simulink model "BLDCmotorControl_FOC_R2017b_fixdt_Ffwd"  (R2017b)
settings: Solver=FixedStepDiscrete  StartTime=0  StopTime=0.5  FixedStep=Ts  MaxStep=1e-6  RelTol=1e-6  AbsTol=1e-6  EnableMultiTasking=on
PreLoadFcn:
  | addpath(genpath('01_Libraries'));
  | addpath(genpath('02_Figures'));
InitFcn:
  | init_model;
values from neighbouring files (symbols this model uses):
  a_elecAngle = 60    [init_model_Ffwd.m]
  b_DCLinkCurrAvail = 0    [init_model_Ffwd.m]
  b_diagEna = 1    [init_model_Ffwd.m]
  b_FfwdEna = 1    [init_model_Ffwd.m]
  b_fieldWeakEna = 0    [init_model_Ffwd.m]
  b_selPhaABCurrMeas = 1    [init_model_Ffwd.m]
  cf_currFilt = 0.02    [init_model_Ffwd.m]
  cf_speedCoef = round(f_ctrl * a_mechAngle * (pi/180) * (30/pi))    [init_model_Ffwd.m]
  cf_speedFilt = 0.20    (= 0.2)    [init_model_Ffwd.m]
  CTRL_COM = 0    [init_model_Ffwd.m]
  dV_openRate = 1000 * Ts_ctrl    (= 0.06)    [init_model_Ffwd.m]
  dz_cntTrnsDetHi = 40    [init_model_Ffwd.m]
  dz_cntTrnsDetLo = 20    [init_model_Ffwd.m]
  i_errThres = 40 * i_sca    (= 2000)    [init_model_Ffwd.m]
  i_max = i_max * i_sca    (= 750)    [init_model_Ffwd.m]
  i_thresOutlier = 200    [init_model_Ffwd.m]
  id_fieldWeak_M1 = [  0   0  0.05  0.25    1    2    3    4  4.5  4.8   5   5] * i_sca    [init_model_Ffwd.m]
  id_Kb = 1000 * Ts_ctrl    (= 0.06)    [init_model_Ffwd.m]
  id_Ki = 80 * Ts_ctrl    (= 0.0048)    [init_model_Ffwd.m]
  id_Kp = 0.5    [init_model_Ffwd.m]
  iq_Kb = 1000 * Ts_ctrl    (= 0.06)    [init_model_Ffwd.m]
  iq_Ki = 100 * Ts_ctrl    (= 0.006)    [init_model_Ffwd.m]
  iq_KiLimProt = 3 * Ts_ctrl    (= 0.00018)    [init_model_Ffwd.m]
  iq_Kp = 0.5    [init_model_Ffwd.m]
  iq_KpLimProt = 4    [init_model_Ffwd.m]
  iq_max_M1 = sqrt(i_max^2 - iq_max_XA.^2)    [init_model_Ffwd.m]
  Ld = 0.00024368    [pe_electric_engine_dyno_data.m]
  Lq = 0.00029758    [pe_electric_engine_dyno_data.m]
  mot_lambda = 0    [init_model_Ffwd.m]
  mot_Ld = 0    [init_model_Ffwd.m]
  mot_Lq = 0    [init_model_Ffwd.m]
  n_commAcvLo = 15    [init_model_Ffwd.m]
  n_commDeacvHi = 30    [init_model_Ffwd.m]
  n_Kb = 1000 * Ts_ctrl    (= 0.06)    [init_model_Ffwd.m]
  n_Ki = 10 * Ts_ctrl    (= 0.0006)    [init_model_Ffwd.m]
  n_Kp = 1    [init_model_Ffwd.m]
  n_KpLimProt = 5    [init_model_Ffwd.m]
  n_max = 800    [init_model_Ffwd.m]
  n_stdStillDet = 3    [init_model_Ffwd.m]
  OPEN_MODE = 0    [init_model_Ffwd.m]
  r_cos_M1 = cos((a_elecAngle_XA + 30)*(pi/180))    [init_model_Ffwd.m]
  r_sin_M1 = sin((a_elecAngle_XA + 30)*(pi/180))    [init_model_Ffwd.m]
  r_whl = 6.5 * 2.54 * 1e-2 / 2    (= 0.08255)    [init_model_Ffwd.m]
  Rs = 0.010087    [pe_electric_engine_dyno_data.m]
  SPD_MODE = 2    [init_model_Ffwd.m]
  t_errDequal = 2 * f_ctrl    (= 32000)    [init_model_Ffwd.m]
  t_errQual = 0.8 * f_ctrl    (= 12800)    [init_model_Ffwd.m]
  TRQ_MODE = 3    [init_model_Ffwd.m]
  Ts = 5e-6    (= 5e-06)    [init_model_Ffwd.m]    (also in pe_electric_engine_dyno_data.m = 1e-05)
  Ts_ctrl = 6e-5    (= 6e-05)    [init_model_Ffwd.m]
  Vd_max = 1000 - V_margin    (= 900)    [init_model_Ffwd.m]
  vec_hallToPos = [0 2 0 1 4 3 5 0]    [init_model_Ffwd.m]
  VLT_MODE = 1    [init_model_Ffwd.m]
  Vq_max_M1 = sqrt(Vd_max^2 - Vq_max_XA.^2)    [init_model_Ffwd.m]
  z_commutMap_M1 = [-1 -1  0  1  1  0 ... (first row only)    [init_model_Ffwd.m]
  z_ctrlModReq = 1    [init_model_Ffwd.m]
  z_ctrlTypSel = 1    [init_model_Ffwd.m]
  z_maxCntRst = 2000    [init_model_Ffwd.m]
undefined symbols (not defined in the file or in its folder): DiscIntNeverNeededParam, sigbuilder_block, V_max, V_min
libraries: powerlib x14, BLDC_controller_Lib x12, simulink x11, pePwmGenerator x1
(part 1 of 3)
Description:
  | This model implements FOC controller for a BLDC motor.
  | The controller is capable for embedded code generation.
  | 
  | Copyright © 2019 Emanuel FERU
settings Model: ExtModeAutoUpdateStatusClock=off  TunableVars=Vd_max,Vq_max_M1,Vq_max_XA,b_DCLinkCurrAvail,b_diagEna,b_fieldWeakEna,b_selPhaABCurrMeas,cf_currFilt,cf_speedCoef,cf_speedFilt,dV_openRate,dz_cntTrnsDetHi,dz_cntTrnsDetLo,i_errThres,i_max,i_thresOutlier,id_Kb,id_Ki,id_Kp,id_fieldWeak_M1,iq_Kb,iq_Ki,iq_KiLimProt,iq_Kp,iq_KpLimProt,iq_max_M1,iq_max_XA,mot_Ld,mot_Lq,mot_lambda,n_Kb,n_Ki,n_Kp,n_KpLimProt,n_commAcvLo,n_commDeacvHi,n_fieldWeak_XA,n_max,n_stdStillDet,t_errDequal,t_errQual,z_ctrlModReq,z_ctrlTypSel,z_maxCntRst  TunableVarsStorageClass=Auto,Auto,Auto,Auto,Auto,Auto,Auto,Auto,Auto,Auto,Auto,Auto,Auto,Auto,Auto,Auto,Auto,Auto,Auto,Auto,Auto,Auto,Auto,Auto,Auto,Auto,Auto,Auto,Auto,Auto,Auto,Auto,Auto,Auto,Auto,Auto,Auto,Auto,Auto,Auto,Auto,Auto,Auto,Auto  TunableVarsTypeQualifier=,,,,,,,,,,,,,,,,,,,,,,,,,,,,,,,,,,,,,,,,,,,  Creator=MathWorks  LastModifiedBy=eferu
settings SolverCC: AutoInsertRateTranBlk=on
settings DataIOCC: LimitDataPoints=on  SaveFormat=Array  ReturnWorkspaceOutputs=on  SignalLoggingName=sigsOut
settings OptimizationCC: DefaultParameterBehavior=Inlined  UseDivisionForNetSlopeComputation=on  UseFloatMulNetSlope=on  UseSpecifiedMinMax=on  InlineInvariantSignals=on  PassReuseOutputArgsAs=Individual arguments  ExpressionDepthLimit=2147483647  ZeroExternalMemoryAtStartup=off  ZeroInternalMemoryAtStartup=off  NoFixptDivByZeroProtection=on  EfficientFloat2IntCast=on  LifeSpan=1  OptimizeBlockOrder=speed  DifferentSizesBufferReuse=on
settings DebuggingCC: ReadBeforeWriteMsg=DisableAll  WriteAfterWriteMsg=DisableAll  WriteAfterReadMsg=DisableAll  UnderspecifiedInitializationDetection=Classic  InheritedTsInSrcMsg=none  MultiTaskDSMMsg=none  MultiTaskCondExecSysMsg=none  ParameterTunabilityLossMsg=error  FcnCallInpInsideContextMsg=warning  StateNameClashWarn=warning  SFUnexpectedBacktrackingDiag=warning  SFNoUnconditionalDefaultTransitionDiag=warning  SFExecutionAtInitializationDiag=none
settings HardwareCC: ProdBitPerPointer=32  ProdBitPerSizeT=32  ProdBitPerPtrDiffT=32  ProdLargestAtomicInteger=Long  ProdLargestAtomicFloat=Double  ProdWordSize=32  ProdHWDeviceType=ARM Compatible->ARM Cortex  TargetUnknown=on
settings ModelReferenceCC: UpdateModelReferenceTargets=IfOutOfDate  PropagateSignalLabelsOutOfModel=off
settings SFSimCC: SFSimEcho=off  MATLABDynamicMemAlloc=off
settings RTWCC: SystemTargetFile=ert.tlc  GenCodeOnly=on  TemplateMakefile=ert_default_tmf  GenerateReport=on  BuildConfiguration=Faster Runs  IncludeHyperlinkInReport=on  LaunchReport=on  GenerateTraceInfo=on  GenerateTraceReport=on  GenerateTraceReportSl=on  GenerateTraceReportSf=on  GenerateTraceReportEml=on  GenerateCodeMetricsReport=on  GenerateCodeReplacementReport=on
settings CodeAppCC: ForceParamTrailComments=on  IgnoreCustomStorageClasses=off  OperatorAnnotations=on  SimulinkDataObjDesc=on  SFDataObjDesc=on  CustomSymbolStrGlobalVar=rt$N$M  CustomSymbolStrType=$N$M  CustomSymbolStrFcn=$N$M$F  CustomSymbolStrMacro=$N$M  InsertBlockDesc=on
settings ERTTargetCC: GenerateSampleERTMain=on  IncludeMdlTerminateFcn=off  CombineSignalStateStructs=on  SuppressErrorStatus=on  MultiInstanceERTCode=on  CodeInterfacePackaging=Reusable function  SupportNonFinite=off  SupportComplex=off  InlinedParameterPlacement=NonHierarchical  RootIOFormat=Part of model data structure  ERTCustomFileTemplate=example_file_process.tlc  ERTFilePackagingFormat=CompactWithDataFile  PreserveStaticInFcnDecls=off
settings ConfigComp: CovMetricSettings=dw  CovHtmlReporting=on  CovSaveCumulativeToWorkspaceVar=on  CovSaveSingleToWorkspaceVar=on  CovExternalEMLEnable=off  CovSFcnEnable=off
settings SimscapeCC: SimscapeNormalizeSystem=off

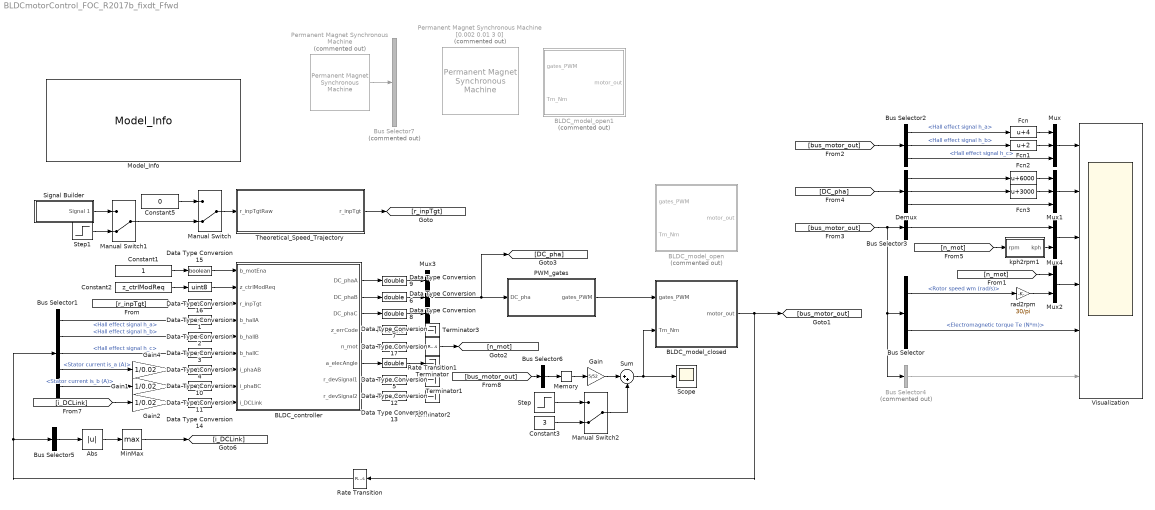
== system BLDCmotorControl_FOC_R2017b_fixdt_Ffwd ==
  Abs : Abs
  BLDC_controller : Subsystem  TreatAsAtomicUnit=on  SystemSampleTime=Ts_ctrl
  BLDC_model_closed : Subsystem
      mask help: Simulink:masks:GenSFuncDesc_MD
      mask Help: eval('feval(''rtwprivate'',''rtwhelpview'',''rtw_sfcn_block'')');
  BLDC_model_open : Subsystem  Commented=on
  BLDC_model_open1 : Subsystem  Commented=on
  Bus Selector : BusSelector  OutputSignals=Rotor speed wm (rad/s),Electromagnetic torque Te (N*m)
  Bus Selector1 : BusSelector  OutputSignals=Hall effect signal h_a,Hall effect signal h_b,Hall effect signal h_c,Stator current is_a (A),Stator current is_b (A)
  Bus Selector2 : BusSelector  OutputSignals=Hall effect signal h_a,Hall effect signal h_b,Hall effect signal h_c
  Bus Selector3 : BusSelector  OutputSignals=Stator current is_a (A),Stator current is_b (A),Stator current is_c (A)  OutputAsBus=on
  Bus Selector4 : BusSelector  Commented=on  OutputSignals=Stator back EMF e_a (V),Stator back EMF e_b (V),Stator back EMF e_cV)  OutputAsBus=on
  Bus Selector5 : BusSelector  OutputSignals=Stator current is_a (A),Stator current is_b (A),Stator current is_c (A)  OutputAsBus=on
  Bus Selector6 : BusSelector  OutputSignals=Rotor speed wm (rad/s)  OutputAsBus=on
  Bus Selector7 : BusSelector  Commented=on  OutputSignals=Hall effect signal h_a,Hall effect signal h_b,Hall effect signal h_c,Stator current is_a (A),Stator current is_b (A)
  Constant1 : Constant  OutDataTypeStr=double
  Constant2 : Constant  Value=z_ctrlModReq  OutDataTypeStr=double
  Constant3 : Constant  Value=3  OutDataTypeStr=double
  Constant5 : Constant  Value=0  OutDataTypeStr=double
  Data Type Conversion{1,10..11,14} (4 alike) : DataTypeConversion  OutDataTypeStr=int16  RndMeth=Zero
  Data Type Conversion{5..9,12..13,17} (8 alike) : DataTypeConversion  OutDataTypeStr=double  RndMeth=Zero
  Data Type Conversion15 : DataTypeConversion  OutDataTypeStr=boolean  RndMeth=Zero
  Data Type Conversion{2..4,16} (4 alike) : DataTypeConversion  OutDataTypeStr=uint8  RndMeth=Zero
  Demux : Demux  Outputs=3
  Fcn : Fcn  Expr=u+4
  Fcn1 : Fcn  Expr=u+2
  Fcn2 : Fcn  Expr=u+6000
  Fcn3 : Fcn  Expr=u+3000
  Gain : Gain  Gain=5/52
  Gain1 : Gain  Tag=struct('comment',struct('text','','placement',1),'logdata',struct('maxnumvals',inf,'plotchannels',[],'loggingmode',3,'channels',1),'output',struct('variable','','description','','name','$S_$B','width',1,'address','','max',NaN,'min',NaN,'class','default','type','CONTINUOUS','scaling','','lsb',1,'offset',0,'arb',0,'freeze',1,'unit','','autoscalingmode',1,'lowerheadroom',1,'upperheadroom',1,'headroomunit','bit','keepdatatype',1,'checkmin',0,'checkmax',0,'castoutput',0,'show',0),'gain',struct('variable','','description','','name','$S_$B_gain','width',1,'address','','max',NaN,'min',NaN,'class','default','type','CONTINUOUS','scaling','','lsb',1,'offset',0,'arb',0,'freeze',1,'unit','','keepdatatype',1,'value','1','scalar',0,'tolerance',1),'scalingvalid',0,'date',730486)  Gain=1/0.02  RndMeth=Zero  SaturateOnIntegerOverflow=on  OutDataTypeStr=Inherit: Same as input  ParamDataTypeStr=Inherit: Same as input
  Gain2 : Gain  Tag=struct('comment',struct('text','','placement',1),'logdata',struct('maxnumvals',inf,'plotchannels',[],'loggingmode',3,'channels',1),'output',struct('variable','','description','','name','$S_$B','width',1,'address','','max',NaN,'min',NaN,'class','default','type','CONTINUOUS','scaling','','lsb',1,'offset',0,'arb',0,'freeze',1,'unit','','autoscalingmode',1,'lowerheadroom',1,'upperheadroom',1,'headroomunit','bit','keepdatatype',1,'checkmin',0,'checkmax',0,'castoutput',0,'show',0),'gain',struct('variable','','description','','name','$S_$B_gain','width',1,'address','','max',NaN,'min',NaN,'class','default','type','CONTINUOUS','scaling','','lsb',1,'offset',0,'arb',0,'freeze',1,'unit','','keepdatatype',1,'value','1','scalar',0,'tolerance',1),'scalingvalid',0,'date',730486)  Gain=1/0.02  RndMeth=Zero  SaturateOnIntegerOverflow=on  OutDataTypeStr=Inherit: Same as input  ParamDataTypeStr=Inherit: Same as input
  Gain4 : Gain  Tag=struct('comment',struct('text','','placement',1),'logdata',struct('maxnumvals',inf,'plotchannels',[],'loggingmode',3,'channels',1),'output',struct('variable','','description','','name','$S_$B','width',1,'address','','max',NaN,'min',NaN,'class','default','type','CONTINUOUS','scaling','','lsb',1,'offset',0,'arb',0,'freeze',1,'unit','','autoscalingmode',1,'lowerheadroom',1,'upperheadroom',1,'headroomunit','bit','keepdatatype',1,'checkmin',0,'checkmax',0,'castoutput',0,'show',0),'gain',struct('variable','','description','','name','$S_$B_gain','width',1,'address','','max',NaN,'min',NaN,'class','default','type','CONTINUOUS','scaling','','lsb',1,'offset',0,'arb',0,'freeze',1,'unit','','keepdatatype',1,'value','1','scalar',0,'tolerance',1),'scalingvalid',0,'date',730486)  Gain=1/0.02  RndMeth=Zero  SaturateOnIntegerOverflow=on  OutDataTypeStr=Inherit: Same as input  ParamDataTypeStr=Inherit: Same as input
  Manual Switch : ManualSwitch  CurrentSetting=0
  Manual Switch1 : ManualSwitch  CurrentSetting=0
  Manual Switch2 : ManualSwitch  CurrentSetting=0
  Memory : Memory
  MinMax : MinMax  Function=max
  Model_Info : BLDC_controller_Lib/Model_Info
  Mux : Mux  Inputs=3
  Mux1 : Mux  Inputs=3
  Mux2 : Mux  Inputs=2
  Mux3 : Mux  Inputs=3
  Mux4 : Mux  Inputs=2
  PWM_gates : Subsystem
  Permanent Magnet Synchronous Machine : powerlib/Machines/Permanent Magnet Synchronous Machine  Commented=on  NbPhases=3  FluxDistribution=Sinusoidal  RotorType=Salient-pole  MechanicalLoad=Torque Tm  PresetModel=No  ShowDetailedParameters=on  MeasurementBus=off  Resistance=0.0485  Inductance=8.5e-3  dqInductances=[8.5e-3,8.5e-3]  La=[0.000395 0.000395]  MachineConstant=Flux linkage established by magnets (V.s)  Flux=0.1194  VoltageCst=86.6271  TorqueCst=0.7164  Flat=120  Mechanical=[0.0027 0.0004924 4 0]  PolePairs=4  InitialConditions=[0,0, 0,0]  InitialConditions5ph=[0 0 0 0 0 0]  TsPowergui=0  TsBlock=-1  RefAngle=90 degrees behind phase A axis (modified Park)
      settings: SourceProductName=Simscape Power Systems
  Permanent Magnet Synchronous Machine [0.002 0.01 3 0] : powerlib/Machines/Permanent Magnet Synchronous Machine  Commented=on  NbPhases=3  FluxDistribution=Sinusoidal  RotorType=Salient-pole  MechanicalLoad=Torque Tm  PresetModel=No  ShowDetailedParameters=on  MeasurementBus=off  Resistance=Rs  Inductance=8.5e-3  dqInductances=[Ld,Lq]  La=0.000395  MachineConstant=Flux linkage established by magnets (V.s)  Flux=Lambda_m  VoltageCst=159.9771  TorqueCst=1.323  Flat=120  Mechanical=[0.0027 0.001 4 0]  PolePairs=Polepairs  InitialConditions=[0,0, 0,0]  InitialConditions5ph=[0 0 0 0 0 0]  TsPowergui=0  TsBlock=-1  RefAngle=Aligned with phase A axis (original Park)
      settings: SourceProductName=Simscape Power Systems
  Rate Transition : RateTransition  Integrity=off  Deterministic=off
  Rate Transition1 : RateTransition  Integrity=off  Deterministic=off
  Scope : Scope
  Signal Builder : Subsystem  Tag=STV Subsys  LoadFcn=sigbuilder_block('load');  StartFcn=sigbuilder_block('start');  StopFcn=sigbuilder_block('stop');  ClipboardFcn=sigbuilder_block('clipboard');  mask(Sigbuilder block){tuvar=[0:10]}
      mask help: Simulink:masks:SigbuilderBlock_MD
      mask init:
      | if ~strcmp(get_param(bdroot(gcbh),'SimulationStatus'),'stopped') tuvar = sigbuilder_block('maskInit'); end
      settings: CopyFcn=sigbuilder_block('copy');  DeleteFcn=sigbuilder_block('delete');  ModelCloseFcn=sigbuilder_block('modelClose');  PreSaveFcn=sigbuilder_block('preSave');  PauseFcn=sigbuilder_block('pause');  ContinueFcn=sigbuilder_block('continue');  NameChangeFcn=sigbuilder_block('namechange');  OpenFcn=sigbuilder_block('open',[141.283 165.057 550.868 400.075 ]);  CloseFcn=sigbuilder_block('close');
      mask Display: plot(0, 0, 100, 100,[2, 2, 32, 32, 2], [68, 8, 8, 68, 68],[32, 2], [38, 38], [32, 19, 2],[53, 60, 44], [32, 17, 17, 2],[16, 16, 31, 31]);txt = getActiveGroup(gcbh);text(2, 100, txt,'verticalAlignment', 'top');
  Step : Step  Time=0.25  Before=-5  After=5  SampleTime=0
  Step1 : Step  Time=0.25  Before=1000  After=-1000
  Sum : Sum  Inputs=|++
  Terminator{,1..3} (4 alike) : Terminator
      settings: Tag=Controls_Lib  Description=Terminator  CopyFcn=Lib_CopyFcn(gcb);  PreDeleteFcn=Lib_PreDeleteFcn(gcb);
  Theoretical_Speed_Trajectory : Subsystem
  Visualization : Scope  NumInputPorts=6
  kph2rpm1 : Subsystem
  rad2rpm : Gain  Gain=30/pi
  wires:
  Mux2/1 -> Visualization/4
  Bus Selector/1 -> rad2rpm/1  "<Rotor speed wm (rad/s)>"
  Bus Selector/2 -> Visualization/5  "<Electromagnetic torque Te (N*m)>"
  Bus Selector2/3 -> Mux/3  "<Hall effect signal h_c>"
  Bus Selector2/2 -> Fcn1/1  "<Hall effect signal h_b>"
  Bus Selector2/1 -> Fcn/1  "<Hall effect signal h_a>"
  Fcn1/1 -> Mux/2
  Mux/1 -> Visualization/1
  Fcn/1 -> Mux/1
  Demux/1 -> Fcn2/1
  Demux/2 -> Fcn3/1
  Fcn2/1 -> Mux1/1
  Fcn3/1 -> Mux1/2
  Demux/3 -> Mux1/3
  Mux1/1 -> Visualization/2
  Bus Selector4/1 -> Visualization/6
  rad2rpm/1 -> Mux2/2
  BLDC_controller/5(n_mot) -> Data Type Conversion7/1
  Sum/1 -> BLDC_model_closed/2(Tm_Nm), Scope/1
  Bus Selector1/2 -> Data Type Conversion3/1  "<Hall effect signal h_b>"
  Bus Selector1/1 -> Data Type Conversion2/1  "<Hall effect signal h_a>"
  Bus Selector1/3 -> Data Type Conversion4/1  "<Hall effect signal h_c>"
  Data Type Conversion2/1 -> BLDC_controller/4("b_hallA ")
  Data Type Conversion3/1 -> BLDC_controller/5(b_hallB)
  Data Type Conversion4/1 -> BLDC_controller/6(b_hallC)
  Theoretical_Speed_Trajectory/1(r_inpTgt) -> [r_inpTgt]
  [r_inpTgt] -> Data Type Conversion1/1
  Data Type Conversion1/1 -> BLDC_controller/3(r_inpTgt)
  BLDC_controller/2(DC_phaB) -> Data Type Conversion6/1
  BLDC_controller/3(DC_phaC) -> Data Type Conversion8/1
  BLDC_controller/1(DC_phaA) -> Data Type Conversion9/1
  Data Type Conversion7/1 -> Rate Transition1/1
  BLDC_controller/6(a_elecAngle) -> Data Type Conversion5/1
  Mux3/1 -> [DC_pha], PWM_gates/1(DC_pha)
  PWM_gates/1(gates_PWM) -> BLDC_model_closed/1(gates_PWM)
  Rate Transition1/1 -> [n_mot]
  [n_mot] -> Mux2/1
  [bus_motor_out] -> Bus Selector2/1
  [bus_motor_out] -> Bus Selector3/1, Bus Selector4/1, Bus Selector/1
  [DC_pha] -> Demux/1
  Manual Switch/1 -> Theoretical_Speed_Trajectory/1(r_inpTgtRaw)
  Constant5/1 -> Manual Switch/1
  Signal Builder/1(Signal 1) -> Manual Switch1/1
  Manual Switch1/1 -> Manual Switch/2
  Step1/1 -> Manual Switch1/2
  Data Type Conversion5/1 -> Terminator/1
  Data Type Conversion8/1 -> Mux3/3
  Data Type Conversion6/1 -> Mux3/2
  Data Type Conversion9/1 -> Mux3/1
  [n_mot] -> kph2rpm1/1(rpm)
  Mux4/1 -> Visualization/3
  Bus Selector3/1 -> Mux4/1
  kph2rpm1/1(kph) -> Mux4/2
  Data Type Conversion10/1 -> BLDC_controller/7(i_phaAB)
  Data Type Conversion11/1 -> BLDC_controller/8(i_phaBC)
  Gain4/1 -> Data Type Conversion10/1
  Gain1/1 -> Data Type Conversion11/1
  BLDC_controller/7(r_devSignal1) -> Data Type Conversion12/1
  Data Type Conversion13/1 -> Terminator2/1
  BLDC_controller/8(r_devSignal2) -> Data Type Conversion13/1
  Gain2/1 -> Data Type Conversion14/1
  Data Type Conversion14/1 -> BLDC_controller/9(i_DCLink)
  [i_DCLink] -> Gain2/1
  Bus Selector1/4 -> Gain4/1  "<Stator current is_a (A)>"
  Bus Selector1/5 -> Gain1/1  "<Stator current is_b (A)>"
  Data Type Conversion15/1 -> BLDC_controller/1(b_motEna)
  Constant1/1 -> Data Type Conversion15/1
  [bus_motor_out] -> Bus Selector6/1
  Bus Selector6/1 -> Memory/1
  Gain/1 -> Sum/1
  Data Type Conversion16/1 -> BLDC_controller/2(z_ctrlModReq)
  Constant2/1 -> Data Type Conversion16/1
  Rate Transition/1 -> Bus Selector1/1, Bus Selector5/1
  Memory/1 -> Gain/1
  Step/1 -> Manual Switch2/1
  Manual Switch2/1 -> Sum/2
  Constant3/1 -> Manual Switch2/2
  Data Type Conversion17/1 -> Terminator3/1
  BLDC_controller/4(z_errCode) -> Data Type Conversion17/1
  Permanent Magnet Synchronous Machine/1 -> Bus Selector7/1
  Data Type Conversion12/1 -> Terminator1/1
  Bus Selector5/1 -> Abs/1
  BLDC_model_closed/1(motor_out) -> Rate Transition/1, [bus_motor_out]
  MinMax/1 -> [i_DCLink]
  Abs/1 -> MinMax/1

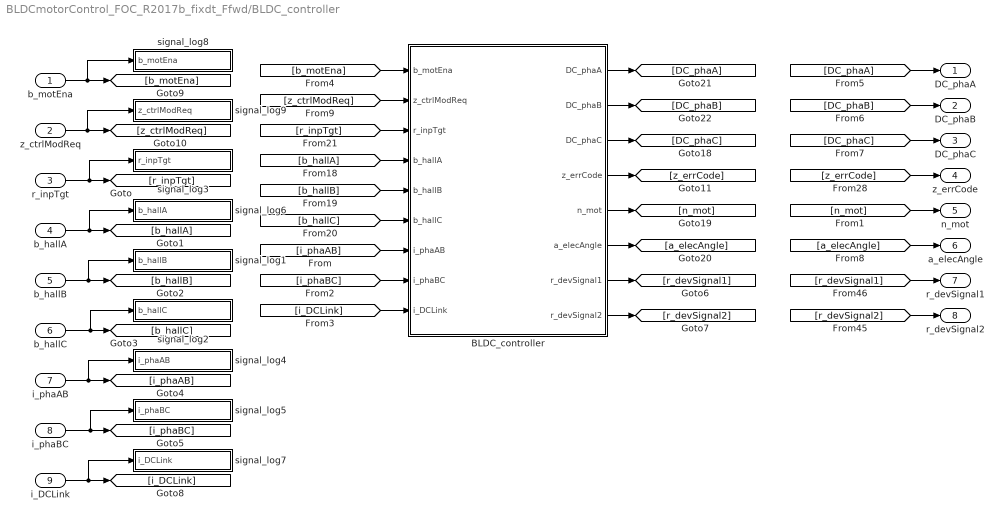
== system BLDCmotorControl_FOC_R2017b_fixdt_Ffwd/BLDC_controller ==
  b_motEna : Inport
  z_ctrlModReq : Inport  Port=2
  r_inpTgt : Inport  Port=3
  "b_hallA " : Inport  Port=4
  b_hallB : Inport  Port=5
  b_hallC : Inport  Port=6
  i_phaAB : Inport  Port=7
  i_phaBC : Inport  Port=8
  i_DCLink : Inport  Port=9
  BLDC_controller : Subsystem  SystemSampleTime=1e-5
  signal_log1 : Subsystem
  signal_log2 : Subsystem
  signal_log3 : Subsystem
  signal_log4 : Subsystem
  signal_log5 : Subsystem
  signal_log6 : Subsystem
  signal_log7 : Subsystem
  signal_log8 : Subsystem
  signal_log9 : Subsystem
  DC_phaA : Outport
  DC_phaB : Outport  Port=2
  DC_phaC : Outport  Port=3
  z_errCode : Outport  Port=4  OutputWhenDisabled=reset  InitialOutput=0
  n_mot : Outport  Port=5
  a_elecAngle : Outport  Port=6
  r_devSignal1 : Outport  Port=7  OutputWhenDisabled=reset  InitialOutput=0
  r_devSignal2 : Outport  Port=8  OutputWhenDisabled=reset  InitialOutput=0
  wires:
  "b_hallA "/1 -> signal_log6/1(b_hallA), [b_hallA]
  b_hallB/1 -> signal_log1/1(b_hallB), [b_hallB]
  b_hallC/1 -> signal_log2/1(b_hallC), [b_hallC]
  [n_mot] -> n_mot/1
  [DC_phaA] -> DC_phaA/1
  [DC_phaB] -> DC_phaB/1
  [DC_phaC] -> DC_phaC/1
  r_inpTgt/1 -> signal_log3/1(r_inpTgt), [r_inpTgt]
  [a_elecAngle] -> a_elecAngle/1
  [r_inpTgt] -> BLDC_controller/3(r_inpTgt)
  [b_hallC] -> BLDC_controller/6(b_hallC)
  [b_hallB] -> BLDC_controller/5(b_hallB)
  [b_hallA] -> BLDC_controller/4("b_hallA ")
  BLDC_controller/6(a_elecAngle) -> [a_elecAngle]
  BLDC_controller/5(n_mot) -> [n_mot]
  BLDC_controller/3(DC_phaC) -> [DC_phaC]
  BLDC_controller/2(DC_phaB) -> [DC_phaB]
  BLDC_controller/1(DC_phaA) -> [DC_phaA]
  i_phaBC/1 -> [i_phaBC], signal_log5/1(i_phaBC)
  i_phaAB/1 -> [i_phaAB], signal_log4/1(i_phaAB)
  [i_phaAB] -> BLDC_controller/7(i_phaAB)
  [i_phaBC] -> BLDC_controller/8(i_phaBC)
  [r_devSignal2] -> r_devSignal2/1
  [r_devSignal1] -> r_devSignal1/1
  BLDC_controller/7(r_devSignal1) -> [r_devSignal1]
  BLDC_controller/8(r_devSignal2) -> [r_devSignal2]
  i_DCLink/1 -> signal_log7/1(i_DCLink), [i_DCLink]
  [i_DCLink] -> BLDC_controller/9(i_DCLink)
  b_motEna/1 -> signal_log8/1(b_motEna), [b_motEna]
  [b_motEna] -> BLDC_controller/1(b_motEna)
  [z_ctrlModReq] -> BLDC_controller/2(z_ctrlModReq)
  z_ctrlModReq/1 -> [z_ctrlModReq], signal_log9/1(z_ctrlModReq)
  [z_errCode] -> z_errCode/1
  BLDC_controller/4(z_errCode) -> [z_errCode]

== system BLDCmotorControl_FOC_R2017b_fixdt_Ffwd/BLDC_model_closed ==
  gates_PWM : Inport
  Tm_Nm : Inport  Port=2
  BLDC_model_sfcn : S-Function  FunctionName=BLDC_model_sf  SFunctionModules=""  SFunctionDeploymentMode=off  EnableBusSupport=off  SFcnStateName=DWORK0  mask{rtw_sf_name=BLDC_model_sf, showVar=off}
      mask prompts: rtw_sf_name "Simulink:masks:GenSFuncName_MP"; showVar "Simulink:masks:GenSFuncShowModuleList_MP"
      mask help: Simulink:masks:GenSFuncDesc_MD
      mask init:
      | displist = '';
      | if ~strcmp(get_param(gcb, 'FunctionName'), rtw_sf_name);
      |   set_param(gcb, 'FunctionName', rtw_sf_name);
      | end
      | % Check if we are generating code
      | rtw_mode = false;
      | if strcmpi(get_param(bdroot(gcb),'SimulationStatus'),'Initializing')
      | 	rtw_mode = strcmpi(get_param(bdroot(gcb),'BuildingRTWCode'),'on') && ...
      | 		~strcmpi(get_param(bdroot(gcb),'TargetStyle'),'SimulationTarget');
      | end
      | if showVar || rtw_mode
      | 	if exist('rtwsfunc') == 2 | exist('rtwsfunc') == 6
      | 		tmplist = rtwsfunc(rtw_sf_name,gcb);
      | 		tmplist = DAStudio.message('Simulink:masks:GenSFuncListOfModules_IC', tmplist);
      | 	elseif showVar
      | 		tmplist1 = DAStudio.message('Simulink:masks:GenSFuncListOfModules_IC', '');
      |         tmplist2 = DAStudio.message('Simulink:masks:GenSFuncNotLicensed_IC');
      |         tmplist = [tmplist1 tmplist2];
      |  	end
      | end
      | if showVar
      |   displist = tmplist;
      | end
      settings: SFcnIsStateOwnerBlock=on
      settings: CopyFcn=|
      | if ~strcmp(get_param(gcb,'Linkstatus'),'none') && ...
      | ~strcmp(get_param(gcb,'Linkstatus'),'implicit')
      |   set_param(gcb,'LinkStatus','none');
      | end
      mask Help: eval('feval(''rtwprivate'',''rtwhelpview'',''rtw_sfcn_block'')');
      mask Display:
      | port_label('input',1,'gates_PWM');
      | port_label('input',2,'Tm_Nm');
      | port_label('output',1,'Stator current is_a (A)');
      | port_label('output',2,'Stator current is_b (A)');
      | port_label('output',3,'Stator current is_c (A)');
      | port_label('output',4,'Stator back EMF e_a (V)');
      | port_label('output',5,'Stator back EMF e_b (V)');
      | port_label('output',6,'Stator back EMF e_cV)');
      | port_label('output',7,'Hall effect signal h_a');
      | port_label('output',8,'Hall effect signal h_b');
      | port_label('output',9,'Hall effect signal h_c');
      | port_label('output',10,'Rotor speed wm (rad/s)');
      | port_label('output',11,'Rotor angle thetam (rad)');
      | port_label('output',12,'Electromagnetic torque Te (N*m)');
  __InputSSForSFun__ : Subsystem
  __OutputSSForSFun__ : Subsystem
  motor_out : Outport
  wires:
  gates_PWM/1 -> __InputSSForSFun__/1(gates_PWM)
  Tm_Nm/1 -> __InputSSForSFun__/2(Tm_Nm)
  __InputSSForSFun__/1(__UniqueOutportName__1__) -> BLDC_model_sfcn/1
  __InputSSForSFun__/2(__UniqueOutportName__2__) -> BLDC_model_sfcn/2
  BLDC_model_sfcn/1 -> __OutputSSForSFun__/1(__UniqueInportName__1__)
  BLDC_model_sfcn/2 -> __OutputSSForSFun__/2(__UniqueInportName__2__)
  BLDC_model_sfcn/3 -> __OutputSSForSFun__/3(__UniqueInportName__3__)
  BLDC_model_sfcn/4 -> __OutputSSForSFun__/4(__UniqueInportName__4__)
  BLDC_model_sfcn/5 -> __OutputSSForSFun__/5(__UniqueInportName__5__)
  BLDC_model_sfcn/6 -> __OutputSSForSFun__/6(__UniqueInportName__6__)
  BLDC_model_sfcn/7 -> __OutputSSForSFun__/7(__UniqueInportName__7__)
  BLDC_model_sfcn/8 -> __OutputSSForSFun__/8(__UniqueInportName__8__)
  BLDC_model_sfcn/9 -> __OutputSSForSFun__/9(__UniqueInportName__9__)
  BLDC_model_sfcn/10 -> __OutputSSForSFun__/10(__UniqueInportName__10__)
  BLDC_model_sfcn/11 -> __OutputSSForSFun__/11(__UniqueInportName__11__)
  BLDC_model_sfcn/12 -> __OutputSSForSFun__/12(__UniqueInportName__12__)
  __OutputSSForSFun__/1(motor_out) -> motor_out/1

== system BLDCmotorControl_FOC_R2017b_fixdt_Ffwd/BLDC_model_open ==
  gates_PWM : Inport
  Tm_Nm : Inport  Port=2
  Constant1 : Constant  Value=36
  Controlled Voltage Source1 : powerlib/Electrical Sources/Controlled Voltage Source  Initialize=on  Source_Type=DC  Amplitude=500  Phase=0  Frequency=0  Measurements=None
  Permanent Magnet Synchronous Machine : powerlib/Machines/Permanent Magnet Synchronous Machine  NbPhases=3  FluxDistribution=Trapezoidal  RotorType=Round  MechanicalLoad=Torque Tm  PresetModel=No  ShowDetailedParameters=on  MeasurementBus=off  Resistance=0.18  Inductance=0.000835  dqInductances=[8.5e-3, 8.5e-3]  La=0.000835  MachineConstant=Flux linkage established by magnets (V.s)  Flux=0.0142879  VoltageCst=44.8868  TorqueCst=0.42864  Flat=120  Mechanical=[0.00621417 0.000303448 15]  PolePairs=15  InitialConditions=[0,0, 0,0]  InitialConditions5ph=[0 0 0 0 0 0]  TsPowergui=0  TsBlock=-1  RefAngle=Aligned with phase A axis (original Park)
      settings: SourceProductName=Simscape Power Systems
  Universal Bridge1 : powerlib/Power Electronics/Universal Bridge  Arms=3  SnubberResistance=5000  SnubberCapacitance=inf  Device=MOSFET / Diodes  Ron=1e-3  Lon=0  ForwardVoltages="[  0  0  ]"  ForwardVoltage=0  GTOparameters=[ 10e-6 , 20e-6 ]  IGBTparameters=[ 1e-6 , 2e-6 ]  Measurements=None  Measurements_2=None  converterType=Rectifier
  Vab : Scope
  Vdc : Scope
  Voltage Measurement : powerlib/Measurements/Voltage Measurement  PhasorSimulation=off  OutputType=Complex  PSBequivalent=0
  Voltage Measurement1 : powerlib/Measurements/Voltage Measurement  PhasorSimulation=off  OutputType=Complex  PSBequivalent=0
  powergui : powerlib/powergui  Priority=2  SimulationMode=Discrete  SampleTime=Ts  frequency=60  Iterations=50  frequencyindice=0  Pbase=100e6  ErrMax=1e-4  UnitsV=kV  UnitsW=MW  buscounter=0  FunctionMessages=off  echomessages=off  EnableUseOfTLC=off  CurrentSourceSwitches=off  DisableSnubberDevices=off  DisableRonSwitches=off  DisableVfSwitches=off  DisplayEquations=off  SolverType=Tustin/Backward Euler (TBE)  Interpol=off  ExternalGateDelay=off  methode=off  Ts=0  x0status=blocks  SPID=off  SwTol=0  HookPort=off  RestoreLinks=warning  ResistiveCurrentMeasurement=off  Frange=[0:2:500]  Ylog=off  Xlog=on  ShowGrid=off  save=off  variable=ZData  structure=0  ZoomFFT=on  StartTime=0.0  cycles=1  DisplayStyle=1  fundamental=60  FreqAxis=off  MaxFrequency=1000  frequencyindicesteady=1  RmsSteady=1  display=off
  motor_out : Outport
  wires:
  Constant1/1 -> Controlled Voltage Source1/1
  Tm_Nm/1 -> Permanent Magnet Synchronous Machine/1
  gates_PWM/1 -> Universal Bridge1/1
  Voltage Measurement1/1 -> Vdc/1
  Permanent Magnet Synchronous Machine/1 -> motor_out/1
  Voltage Measurement/1 -> Vab/1
  connections:
  Voltage Measurement/LConn2 -- Permanent Magnet Synchronous Machine/LConn2 -- Universal Bridge1/LConn2
  Voltage Measurement1/LConn1 -- Controlled Voltage Source1/RConn1 -- Universal Bridge1/RConn1
  Universal Bridge1/RConn2 -- Controlled Voltage Source1/LConn1 -- Voltage Measurement1/LConn2
  Universal Bridge1/LConn3 -- Permanent Magnet Synchronous Machine/LConn3
  Universal Bridge1/LConn1 -- Permanent Magnet Synchronous Machine/LConn1 -- Voltage Measurement/LConn1

== system BLDCmotorControl_FOC_R2017b_fixdt_Ffwd/BLDC_model_open1 ==
  gates_PWM : Inport
  Tm_Nm : Inport  Port=2
  Constant1 : Constant  Value=36
  Controlled Voltage Source1 : powerlib/Electrical Sources/Controlled Voltage Source  Initialize=on  Source_Type=DC  Amplitude=500  Phase=0  Frequency=0  Measurements=None
  Permanent Magnet Synchronous Machine : powerlib/Machines/Permanent Magnet Synchronous Machine  NbPhases=3  FluxDistribution=Sinusoidal  RotorType=Salient-pole  MechanicalLoad=Torque Tm  PresetModel=No  ShowDetailedParameters=on  MeasurementBus=off  Resistance=0.15  Inductance=0.000835  dqInductances=[1.5e-3, 3.5e-3]  La=0.000835  MachineConstant=Flux linkage established by magnets (V.s)  Flux=0.0442879  VoltageCst=120.494  TorqueCst=0.99648  Flat=120  Mechanical=[10*1.9089e-4 0.0303448 15]  PolePairs=15  InitialConditions=[0,0, 0,0]  InitialConditions5ph=[0 0 0 0 0 0]  TsPowergui=0  TsBlock=-1  RefAngle=Aligned with phase A axis (original Park)
      settings: SourceProductName=Simscape Power Systems
  Universal Bridge1 : powerlib/Power Electronics/Universal Bridge  Arms=3  SnubberResistance=5000  SnubberCapacitance=inf  Device=MOSFET / Diodes  Ron=1e-3  Lon=0  ForwardVoltages="[  0  0  ]"  ForwardVoltage=0  GTOparameters=[ 10e-6 , 20e-6 ]  IGBTparameters=[ 1e-6 , 2e-6 ]  Measurements=None  Measurements_2=None  converterType=Rectifier
  Vab : Scope
  Vdc : Scope
  Voltage Measurement : powerlib/Measurements/Voltage Measurement  PhasorSimulation=off  OutputType=Complex  PSBequivalent=0
  Voltage Measurement1 : powerlib/Measurements/Voltage Measurement  PhasorSimulation=off  OutputType=Complex  PSBequivalent=0
  powergui : powerlib/powergui  Priority=2  SimulationMode=Discrete  SampleTime=Ts  frequency=60  Iterations=50  frequencyindice=0  Pbase=100e6  ErrMax=1e-4  UnitsV=kV  UnitsW=MW  buscounter=0  FunctionMessages=off  echomessages=off  EnableUseOfTLC=off  CurrentSourceSwitches=off  DisableSnubberDevices=off  DisableRonSwitches=off  DisableVfSwitches=off  DisplayEquations=off  SolverType=Tustin/Backward Euler (TBE)  Interpol=off  ExternalGateDelay=off  methode=off  Ts=0  x0status=blocks  SPID=off  SwTol=0  HookPort=off  RestoreLinks=warning  ResistiveCurrentMeasurement=off  Frange=[0:2:500]  Ylog=off  Xlog=on  ShowGrid=off  save=off  variable=ZData  structure=0  ZoomFFT=on  StartTime=0.0  cycles=1  DisplayStyle=1  fundamental=60  FreqAxis=off  MaxFrequency=1000  frequencyindicesteady=1  RmsSteady=1  display=off
  motor_out : Outport
  wires:
  Voltage Measurement/1 -> Vab/1
  Permanent Magnet Synchronous Machine/1 -> motor_out/1
  Voltage Measurement1/1 -> Vdc/1
  gates_PWM/1 -> Universal Bridge1/1
  Tm_Nm/1 -> Permanent Magnet Synchronous Machine/1
  Constant1/1 -> Controlled Voltage Source1/1
  connections:
  Voltage Measurement/LConn1 -- Permanent Magnet Synchronous Machine/LConn1 -- Universal Bridge1/LConn1
  Universal Bridge1/LConn3 -- Permanent Magnet Synchronous Machine/LConn3
  Voltage Measurement1/LConn2 -- Controlled Voltage Source1/LConn1 -- Universal Bridge1/RConn2
  Universal Bridge1/RConn1 -- Controlled Voltage Source1/RConn1 -- Voltage Measurement1/LConn1
  Universal Bridge1/LConn2 -- Permanent Magnet Synchronous Machine/LConn2 -- Voltage Measurement/LConn2

== system BLDCmotorControl_FOC_R2017b_fixdt_Ffwd/PWM_gates ==
  DC_pha : Inport
  Abs : Abs  OutDataTypeStr=Inherit: Inherit via back propagation  RndMeth=Zero
  Abs1 : Abs  OutDataTypeStr=Inherit: Inherit via back propagation  RndMeth=Zero
  Abs2 : Abs  OutDataTypeStr=Inherit: Inherit via back propagation  RndMeth=Zero
  Constant4 : Constant  Value=0  OutDataTypeStr=Inherit: Inherit via back propagation
  Demux : Demux  Outputs=3
  Gain8 : Gain  Gain=1/1000  OutDataTypeStr=Inherit: Inherit via back propagation  RndMeth=Zero
  MinMax : MinMax  Inputs=2  OutDataTypeStr=Inherit: Inherit via back propagation  RndMeth=Zero
  MinMax1 : MinMax  Function=max  Inputs=2  OutDataTypeStr=Inherit: Inherit via back propagation  RndMeth=Zero
  MinMax2 : MinMax  Inputs=2  OutDataTypeStr=Inherit: Inherit via back propagation  RndMeth=Zero
  MinMax3 : MinMax  Function=max  Inputs=2  OutDataTypeStr=Inherit: Inherit via back propagation  RndMeth=Zero
  MinMax4 : MinMax  Inputs=2  OutDataTypeStr=Inherit: Inherit via back propagation  RndMeth=Zero
  MinMax5 : MinMax  Function=max  Inputs=2  OutDataTypeStr=Inherit: Inherit via back propagation  RndMeth=Zero
  Mux4 : Mux  Inputs=6
  PWM_generator : pePwmGenerator/PWM Generator  Commented=on  CarrCount=Up  Tper=5e-5  Ts=5e-6
      settings: SourceProductName=The database C:\Users\37ef\AppData\Roaming\MathWorks\MATLAB\R2017b\slblocks_master.db is locked, or a table in the database is locked. (database is locked)
  PWM_generator1 : Subsystem
      mask help: Simulink:masks:GenSFuncDesc_MD
      mask Help: eval('feval(''rtwprivate'',''rtwhelpview'',''rtw_sfcn_block'')');
  PWM_generator12 : Subsystem
      mask help: Simulink:masks:GenSFuncDesc_MD
      mask Help: eval('feval(''rtwprivate'',''rtwhelpview'',''rtw_sfcn_block'')');
  PWM_generator2 : Subsystem
      mask help: Simulink:masks:GenSFuncDesc_MD
      mask Help: eval('feval(''rtwprivate'',''rtwhelpview'',''rtw_sfcn_block'')');
  PWM_generator3 : Subsystem
      mask help: Simulink:masks:GenSFuncDesc_MD
      mask Help: eval('feval(''rtwprivate'',''rtwhelpview'',''rtw_sfcn_block'')');
  PWM_generator4 : Subsystem
      mask help: Simulink:masks:GenSFuncDesc_MD
      mask Help: eval('feval(''rtwprivate'',''rtwhelpview'',''rtw_sfcn_block'')');
  PWM_generator5 : Subsystem
      mask help: Simulink:masks:GenSFuncDesc_MD
      mask Help: eval('feval(''rtwprivate'',''rtwhelpview'',''rtw_sfcn_block'')');
  signal_log6 : Subsystem
  gates_PWM : Outport
  wires:
  PWM_generator4/1(PWM) -> Mux4/5
  Abs/1 -> PWM_generator1/1(DC)
  PWM_generator12/1(PWM) -> Mux4/1
  PWM_generator5/1(PWM) -> Mux4/6
  MinMax1/1 -> PWM_generator12/1(DC)
  PWM_generator3/1(PWM) -> Mux4/4
  PWM_generator1/1(PWM) -> Mux4/2
  MinMax5/1 -> PWM_generator4/1(DC)
  PWM_generator2/1(PWM) -> Mux4/3
  Abs2/1 -> PWM_generator5/1(DC)
  MinMax3/1 -> PWM_generator2/1(DC)
  Abs1/1 -> PWM_generator3/1(DC)
  Demux/1 -> MinMax/2, MinMax1/2
  MinMax4/1 -> Abs2/1
  Constant4/1 -> MinMax1/1, MinMax4/1, MinMax5/1, MinMax2/1, MinMax3/1, MinMax/1
  MinMax2/1 -> Abs1/1
  Demux/2 -> MinMax2/2, MinMax3/2
  MinMax/1 -> Abs/1
  Demux/3 -> MinMax5/2, MinMax4/2
  DC_pha/1 -> Gain8/1
  Gain8/1 -> Demux/1
  Mux4/1 -> signal_log6/1(PWM), gates_PWM/1

== system BLDCmotorControl_FOC_R2017b_fixdt_Ffwd/Signal Builder ==
  Demux : Demux  Tag=STV Demux  Outputs=1
  FromWs : FromWorkspace  Tag=STV FromWs  VariableName=tuvar
      SigBuilderData=|
      | common.afterFinalStr = 'Extrapolate'
      | common.sampleTime = '-1'
      | dataSet.timeRange = [0 1.5]
      | dataSet.name = 'Group 1'
      | sbobj.Groups.Name = 'Group 1'
      | sbobj.Groups.Signals.Name = 'Signal 1'
      | sbobj.Groups.Signals.XData = [0 0.2 0.4 0.6 0.8 1.5]
      | sbobj.Groups.Signals.YData = [0 800 800 600 -800 -800]
      | sbobj.Groups.TimeRange = [0 1.5]
  Signal 1 : Outport  Tag=STV Outport
  wires:
  Demux/1 -> Signal 1/1
  FromWs/1 -> Demux/1

== system BLDCmotorControl_FOC_R2017b_fixdt_Ffwd/Theoretical_Speed_Trajectory ==
  note: Ideal Speed Trajectory Calculation
      | Based on Min/Max torque and Min/Max torque rate constraints
  r_inpTgtRaw : Inport
  Discrete Derivative1 : simulink/Discrete/Discrete Derivative  gainval=1.0  ICPrevScaledInput=0.0  OutMin=[]  OutMax=[]  OutDataType=fixdt(1, 16)  OutScaling=2^-10  DoSatur=off
  Discrete Derivative2 : simulink/Discrete/Discrete Derivative  gainval=1.0  ICPrevScaledInput=0.0  OutMin=[]  OutMax=[]  OutDataType=fixdt(1, 16)  OutScaling=2^-10  DoSatur=off
  Discrete-Time Integrator2 : DiscreteIntegrator  SampleTime=-1  ICPrevOutput=DiscIntNeverNeededParam  ICPrevScaledInput=DiscIntNeverNeededParam
  Divide2 : Product  Inputs=*/
  Divide3 : Product  Inputs=**
  Divide4 : Product  Inputs=**
  Gain1 : Gain  Gain=-1
  Gain2 : Gain  Gain=-1
  Gain4 : Gain  Gain=pi/30
  Gain5 : Gain  Gain=30/pi
  J_mot : Constant  Value=0.01  OutDataTypeStr=Inherit: Inherit via back propagation
  Kp : Constant  Value=65  OutDataTypeStr=Inherit: Inherit via back propagation
  M_max : Constant  Value=15  OutDataTypeStr=Inherit: Inherit via back propagation
  Manual Switch : ManualSwitch
  Mux4 : Mux  Inputs=2
  Rate Limiter Dynamic3 : simulink/Discontinuities/Rate Limiter Dynamic
      settings: SourceProductName=Simulink
  Saturation Dynamic : simulink/Discontinuities/Saturation Dynamic  OutMin=[]  OutMax=[]  OutDataTypeStr=Inherit: Same as second input  OutDataType=fixdt(1, 16)  OutScaling=2^-10  DoSatur=off
  Scope : Scope  NumInputPorts=3
  Sum2 : Sum  Inputs=|+-  RndMeth=Zero  OutDataTypeStr=Inherit: Same as first input
  Sum8 : Sum  Inputs=++|  RndMeth=Zero  OutDataTypeStr=Inherit: Same as first input
  dM_max : Constant  Value=500  OutDataTypeStr=Inherit: Inherit via back propagation
  r_inpTgt : Outport
  wires:
  Gain4/1 -> Divide4/2  "dw"
  M_max/1 -> Gain1/1, Saturation Dynamic/1
  J_mot/1 -> Divide2/2, Divide4/1
  Divide2/1 -> Gain5/1  "w"
  [r_inpTgtRaw] -> Discrete Derivative2/1, Sum2/1
  Divide4/1 -> Saturation Dynamic/2  "M"
  Gain1/1 -> Saturation Dynamic/3
  dM_max/1 -> Gain2/1, Rate Limiter Dynamic3/1
  Sum2/1 -> Divide3/2
  Divide3/1 -> Sum8/2
  Rate Limiter Dynamic3/1 -> [M_tgtTheo], Discrete-Time Integrator2/1
  Gain2/1 -> Rate Limiter Dynamic3/3
  Sum8/1 -> Gain4/1  "dn"
  Saturation Dynamic/1 -> Rate Limiter Dynamic3/2
  Gain5/1 -> [r_inpTgt], Sum2/2  "rpm"
  Kp/1 -> Divide3/1
  Discrete-Time Integrator2/1 -> Divide2/1
  Mux4/1 -> Scope/1
  Discrete Derivative1/1 -> Scope/3
  Discrete Derivative2/1 -> Sum8/1
  [M_tgtTheo] -> Discrete Derivative1/1, Scope/2
  r_inpTgtRaw/1 -> [r_inpTgtRaw]
  [r_inpTgtRaw] -> Mux4/1
  [r_inpTgt] -> Mux4/2
  [r_inpTgt] -> Manual Switch/2
  Manual Switch/1 -> r_inpTgt/1
  [r_inpTgtRaw] -> Manual Switch/1

== system BLDCmotorControl_FOC_R2017b_fixdt_Ffwd/kph2rpm1 ==
  rpm : Inport
  Divide2 : Product  Inputs=**  RndMeth=Zero  OutDataTypeStr=Inherit: Same as first input
  Gain4 : Gain  Gain=pi/30  RndMeth=Zero  OutDataTypeStr=Inherit: Same as input
  Gain5 : Gain  Gain=3.6  RndMeth=Zero  OutDataTypeStr=Inherit: Same as input
  const2 : Constant  Value=r_whl  OutDataTypeStr=Inherit: Inherit via back propagation
  kph : Outport
  wires:
  rpm/1 -> Gain4/1
  Gain4/1 -> Divide2/1  "radps"
  const2/1 -> Divide2/2
  Divide2/1 -> Gain5/1  "mps"
  Gain5/1 -> kph/1

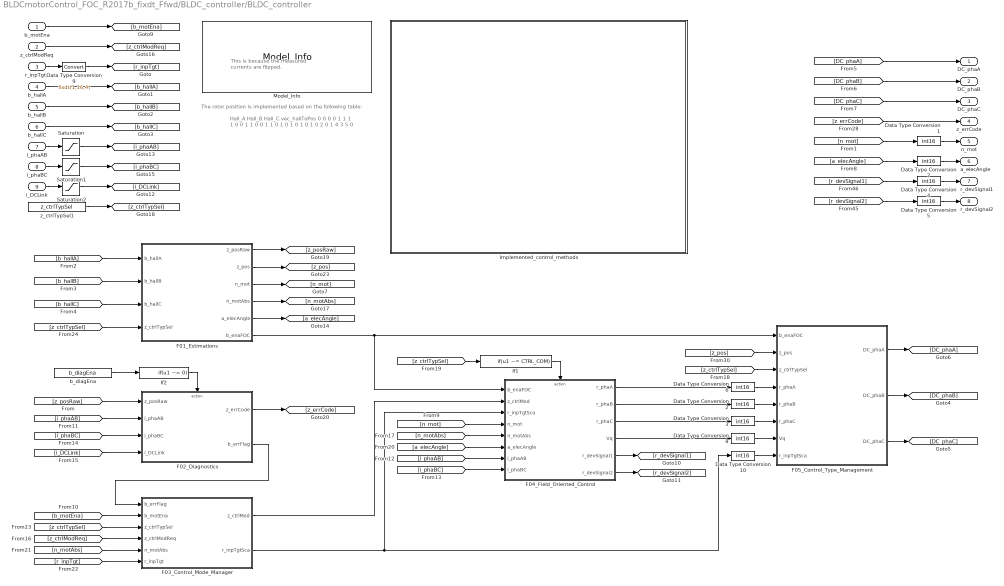
== system BLDCmotorControl_FOC_R2017b_fixdt_Ffwd/BLDC_controller/BLDC_controller ==
  note: The rotor position is implemented based on the following table:
  note: Hall_A
      | Hall_B
      | Hall_C
      | vec_hallToPos
      |
      | 0
      | 0
      | 0
      | 0
      | 1
      | 1
      | 1
      | 1
      | 0
      | 0
      | 1
      | 1
      | 0
      | 0
      | 1
      | 1
      | 0
      | 1
      | 0
      | 1
      | 0
      | 1
      | 0
      | 1
      | 0
      | 2
      | 0
      | 1
      | 4
      | 3
      | 5
      | 0
  note: This is because the measured currents are flipped.
  b_motEna : Inport
  z_ctrlModReq : Inport  Port=2
  r_inpTgt : Inport  Port=3
  "b_hallA " : Inport  Port=4
  b_hallB : Inport  Port=5
  b_hallC : Inport  Port=6
  i_phaAB : Inport  Port=7
  i_phaBC : Inport  Port=8
  i_DCLink : Inport  Port=9
  Data Type Conversion{1..8,10} (9 alike) : DataTypeConversion  OutDataTypeStr=int16
  Data Type Conversion9 : DataTypeConversion  OutDataTypeStr=fixdt(1,16,4)
  F01_Estimations : Subsystem
  F02_Diagnostics : Subsystem
  F03_Control_Mode_Manager : Subsystem
  F04_Field_Oriented_Control : Subsystem
  F05_Control_Type_Management : Subsystem
  If1 : If  IfExpression=u1 ~= CTRL_COM  ShowElse=off
  If2 : If  IfExpression=u1 ~= 0  ShowElse=off
  Implemented_control_methods : Subsystem
      mask Display: image('control_methods.png')
  Model_Info : BLDC_controller_Lib/Model_Info
  Saturation : Saturate  UpperLimit=1500  LowerLimit=-1500  OutDataTypeStr=fixdt(1,16,4)
  Saturation1 : Saturate  UpperLimit=1500  LowerLimit=-1500  OutDataTypeStr=fixdt(1,16,4)
  Saturation2 : Saturate  UpperLimit=1500  LowerLimit=-1500  OutDataTypeStr=fixdt(1,16,4)
  b_diagEna : Constant  Value=b_diagEna  OutDataTypeStr=boolean
  z_ctrlTypSel1 : Constant  Value=z_ctrlTypSel  OutDataTypeStr=uint8
  DC_phaA : Outport
  DC_phaB : Outport  Port=2
  DC_phaC : Outport  Port=3
  z_errCode : Outport  Port=4  OutputWhenDisabled=reset  InitialOutput=0
  n_mot : Outport  Port=5
  a_elecAngle : Outport  Port=6
  r_devSignal1 : Outport  Port=7  OutputWhenDisabled=reset  InitialOutput=0
  r_devSignal2 : Outport  Port=8  OutputWhenDisabled=reset  InitialOutput=0
  wires:
  "b_hallA "/1 -> [b_hallA]
  b_hallB/1 -> [b_hallB]
  b_hallC/1 -> [b_hallC]
  [n_mot] -> Data Type Conversion1/1
  [DC_phaA] -> DC_phaA/1
  [b_hallA] -> F01_Estimations/1(b_hallA)
  [b_hallC] -> F01_Estimations/3(b_hallC)
  [b_hallB] -> F01_Estimations/2(b_hallB)
  F01_Estimations/3("n_mot ") -> [n_mot]
  F04_Field_Oriented_Control/1(r_phaA) -> Data Type Conversion6/1
  F04_Field_Oriented_Control/2(r_phaB) -> Data Type Conversion2/1
  F04_Field_Oriented_Control/3("r_phaC ") -> Data Type Conversion3/1
  Data Type Conversion8/1 -> F05_Control_Type_Management/7(Vq)
  F05_Control_Type_Management/1(DC_phaA) -> [DC_phaA]
  F05_Control_Type_Management/2(DC_phaB) -> [DC_phaB]
  F05_Control_Type_Management/3("DC_phaC ") -> [DC_phaC]
  [DC_phaB] -> DC_phaB/1
  [DC_phaC] -> DC_phaC/1
  r_inpTgt/1 -> Data Type Conversion9/1
  [a_elecAngle] -> Data Type Conversion7/1
  Data Type Conversion6/1 -> F05_Control_Type_Management/4(r_phaA)
  Data Type Conversion2/1 -> F05_Control_Type_Management/5(r_phaB)
  Data Type Conversion3/1 -> F05_Control_Type_Management/6(r_phaC)
  [i_phaBC] -> F04_Field_Oriented_Control/8(i_phaBC)
  [i_phaAB] -> F04_Field_Oriented_Control/7(i_phaAB)
  i_phaAB/1 -> Saturation/1
  i_phaBC/1 -> Saturation1/1
  F04_Field_Oriented_Control/5(r_devSignal1) -> [r_devSignal1]
  [i_DCLink] -> F02_Diagnostics/4(i_DCLink)
  i_DCLink/1 -> Saturation2/1
  F04_Field_Oriented_Control/4(Vq) -> Data Type Conversion8/1
  Data Type Conversion9/1 -> [r_inpTgt]
  Saturation/1 -> [i_phaAB]
  Saturation1/1 -> [i_phaBC]
  Saturation2/1 -> [i_DCLink]
  [n_mot] -> F04_Field_Oriented_Control/4(n_mot)
  b_motEna/1 -> [b_motEna]
  [b_motEna] -> F03_Control_Mode_Manager/2(b_motEna)
  F04_Field_Oriented_Control/6(r_devSignal2) -> [r_devSignal2]
  Data Type Conversion1/1 -> n_mot/1
  F01_Estimations/5(a_elecAngle) -> [a_elecAngle]
  Data Type Conversion7/1 -> a_elecAngle/1
  [z_ctrlModReq] -> F03_Control_Mode_Manager/4(z_ctrlModReq)
  z_ctrlModReq/1 -> [z_ctrlModReq]
  F01_Estimations/4(n_motAbs) -> [n_motAbs]
  [n_motAbs] -> F04_Field_Oriented_Control/5(n_motAbs)
  F03_Control_Mode_Manager/2(r_inpTgtSca) -> F04_Field_Oriented_Control/3(r_inpTgtSca), Data Type Conversion10/1
  Data Type Conversion10/1 -> F05_Control_Type_Management/8(r_inpTgtSca)
  [z_ctrlTypSel] -> F05_Control_Type_Management/3(z_ctrlTypSel)
  [z_ctrlTypSel] -> If1/1
  [a_elecAngle] -> F04_Field_Oriented_Control/6(a_elecAngle)
  [n_motAbs] -> F03_Control_Mode_Manager/5(n_motAbs)
  [r_inpTgt] -> F03_Control_Mode_Manager/6(r_inpTgt)
  [z_ctrlTypSel] -> F03_Control_Mode_Manager/3(z_ctrlTypSel)
  z_ctrlTypSel1/1 -> [z_ctrlTypSel]
  [z_ctrlTypSel] -> F01_Estimations/4(z_ctrlTypSel)
  If2/1 -> F02_Diagnostics/Action
  F01_Estimations/1(z_posRaw) -> [z_posRaw]
  [z_posRaw] -> F02_Diagnostics/1(z_posRaw)
  F02_Diagnostics/1("z_errCode ") -> [z_errCode]
  b_diagEna/1 -> If2/1
  [z_errCode] -> z_errCode/1
  F03_Control_Mode_Manager/1(z_ctrlMod) -> F04_Field_Oriented_Control/2(z_ctrlMod)
  F01_Estimations/2(z_pos) -> [z_pos]
  [z_pos] -> F05_Control_Type_Management/2(z_pos)
  F01_Estimations/6(b_enaFOC) -> F05_Control_Type_Management/1(b_enaFOC), F04_Field_Oriented_Control/1(b_enaFOC)
  [r_devSignal1] -> Data Type Conversion4/1
  [r_devSignal2] -> Data Type Conversion5/1
  F02_Diagnostics/2(b_errFlag) -> F03_Control_Mode_Manager/1(b_errFlag)
  If1/1 -> F04_Field_Oriented_Control/Action
  Data Type Conversion4/1 -> r_devSignal1/1
  Data Type Conversion5/1 -> r_devSignal2/1
  [i_phaAB] -> F02_Diagnostics/2(i_phaAB)
  [i_phaBC] -> F02_Diagnostics/3(i_phaBC)

== system BLDCmotorControl_FOC_R2017b_fixdt_Ffwd/BLDC_controller/signal_log1 ==
  b_hallB : Inport
  Terminator_1 : Terminator
  wires:
  b_hallB/1 -> Terminator_1/1  "b_hallB"

== system BLDCmotorControl_FOC_R2017b_fixdt_Ffwd/BLDC_controller/signal_log2 ==
  b_hallC : Inport
  Terminator_1 : Terminator
  wires:
  b_hallC/1 -> Terminator_1/1  "b_hallC"

== system BLDCmotorControl_FOC_R2017b_fixdt_Ffwd/BLDC_controller/signal_log3 ==
  r_inpTgt : Inport
  Terminator_1 : Terminator
  wires:
  r_inpTgt/1 -> Terminator_1/1  "r_inpTgt"

== system BLDCmotorControl_FOC_R2017b_fixdt_Ffwd/BLDC_controller/signal_log4 ==
  i_phaAB : Inport
  Terminator_1 : Terminator
  wires:
  i_phaAB/1 -> Terminator_1/1  "i_phaAB"

== system BLDCmotorControl_FOC_R2017b_fixdt_Ffwd/BLDC_controller/signal_log5 ==
  i_phaBC : Inport
  Terminator_1 : Terminator
  wires:
  i_phaBC/1 -> Terminator_1/1  "i_phaBC"

== system BLDCmotorControl_FOC_R2017b_fixdt_Ffwd/BLDC_controller/signal_log6 ==
  b_hallA : Inport
  Terminator_1 : Terminator
  wires:
  b_hallA/1 -> Terminator_1/1  "b_hallA"

== system BLDCmotorControl_FOC_R2017b_fixdt_Ffwd/BLDC_controller/signal_log7 ==
  i_DCLink : Inport
  Terminator_1 : Terminator
  wires:
  i_DCLink/1 -> Terminator_1/1  "i_DCLink"

== system BLDCmotorControl_FOC_R2017b_fixdt_Ffwd/BLDC_controller/signal_log8 ==
  b_motEna : Inport
  Terminator_1 : Terminator
  wires:
  b_motEna/1 -> Terminator_1/1  "b_motEna"

== system BLDCmotorControl_FOC_R2017b_fixdt_Ffwd/BLDC_controller/signal_log9 ==
  z_ctrlModReq : Inport
  Terminator_1 : Terminator
  wires:
  z_ctrlModReq/1 -> Terminator_1/1  "z_ctrlModReq"

== system BLDCmotorControl_FOC_R2017b_fixdt_Ffwd/BLDC_model_closed/__InputSSForSFun__ ==
  gates_PWM : Inport
  Tm_Nm : Inport  Port=2
  __UniqueOutportName__1__ : Outport
  __UniqueOutportName__2__ : Outport  Port=2
  wires:
  gates_PWM/1 -> __UniqueOutportName__1__/1
  Tm_Nm/1 -> __UniqueOutportName__2__/1

== system BLDCmotorControl_FOC_R2017b_fixdt_Ffwd/BLDC_model_closed/__OutputSSForSFun__ ==
  __UniqueInportName__1__ : Inport
  __UniqueInportName__2__ : Inport  Port=2
  __UniqueInportName__3__ : Inport  Port=3
  __UniqueInportName__4__ : Inport  Port=4
  __UniqueInportName__5__ : Inport  Port=5
  __UniqueInportName__6__ : Inport  Port=6
  __UniqueInportName__7__ : Inport  Port=7
  __UniqueInportName__8__ : Inport  Port=8
  __UniqueInportName__9__ : Inport  Port=9
  __UniqueInportName__10__ : Inport  Port=10
  __UniqueInportName__11__ : Inport  Port=11
  __UniqueInportName__12__ : Inport  Port=12
  Mux1 : BusCreator  Inputs=12
  motor_out : Outport
  wires:
  __UniqueInportName__1__/1 -> Mux1/1  "Stator current is_a (A)"
  __UniqueInportName__2__/1 -> Mux1/2  "Stator current is_b (A)"
  __UniqueInportName__3__/1 -> Mux1/3  "Stator current is_c (A)"
  __UniqueInportName__4__/1 -> Mux1/4  "Stator back EMF e_a (V)"
  __UniqueInportName__5__/1 -> Mux1/5  "Stator back EMF e_b (V)"
  __UniqueInportName__6__/1 -> Mux1/6  "Stator back EMF e_cV)"
  __UniqueInportName__7__/1 -> Mux1/7  "Hall effect signal h_a"
  __UniqueInportName__8__/1 -> Mux1/8  "Hall effect signal h_b"
  __UniqueInportName__9__/1 -> Mux1/9  "Hall effect signal h_c"
  __UniqueInportName__10__/1 -> Mux1/10  "Rotor speed wm (rad/s)"
  __UniqueInportName__11__/1 -> Mux1/11  "Rotor angle thetam (rad)"
  __UniqueInportName__12__/1 -> Mux1/12  "Electromagnetic torque Te (N*m)"
  Mux1/1 -> motor_out/1

== system BLDCmotorControl_FOC_R2017b_fixdt_Ffwd/PWM_gates/PWM_generator1 ==
  DC : Inport  SampleTime=Ts
  PWM_generator_sfcn : S-Function  FunctionName=PWM_generator_sf  SFunctionModules=""  SFunctionDeploymentMode=off  EnableBusSupport=off  SFcnStateName=DWORK0  mask{rtw_sf_name=PWM_generator_sf, showVar=off}
      mask prompts: rtw_sf_name "Simulink:masks:GenSFuncName_MP"; showVar "Simulink:masks:GenSFuncShowModuleList_MP"
      mask help: Simulink:masks:GenSFuncDesc_MD
      mask init: same as BLDCmotorControl_FOC_R2017b_fixdt_Ffwd/BLDC_model_closed/BLDC_model_sfcn
      settings: SFcnIsStateOwnerBlock=on
      settings: CopyFcn=|
      | if ~strcmp(get_param(gcb,'Linkstatus'),'none') && ...
      | ~strcmp(get_param(gcb,'Linkstatus'),'implicit')
      |   set_param(gcb,'LinkStatus','none');
      | end
      mask Help: eval('feval(''rtwprivate'',''rtwhelpview'',''rtw_sfcn_block'')');
      mask Display:
      | port_label('input',1,'DC');
      | port_label('output',1,'PWM');
  __InputSSForSFun__ : Subsystem
  __OutputSSForSFun__ : Subsystem
  PWM : Outport
  wires:
  __OutputSSForSFun__/1(PWM) -> PWM/1
  PWM_generator_sfcn/1 -> __OutputSSForSFun__/1(__UniqueInportName__1__)
  __InputSSForSFun__/1(__UniqueOutportName__1__) -> PWM_generator_sfcn/1
  DC/1 -> __InputSSForSFun__/1(DC)
